simulink model "PCH_660_400_x3_6arm"  (R2018b)
settings: Solver=ode23t  StartTime=0.0  StopTime=0.1  RelTol=1e-3
undefined symbols (not defined in the file): C_load, fn, L_load, L_load1, R12pu, R_load, Rmpu, Stv, U1, U2, X12pu, Xmpu
libraries: powerlib x82, powerlib_meascontrol x27, peRmsMeasurement x17
(part 1 of 2)
settings Model: Creator=K2  LastModifiedBy=VID Company

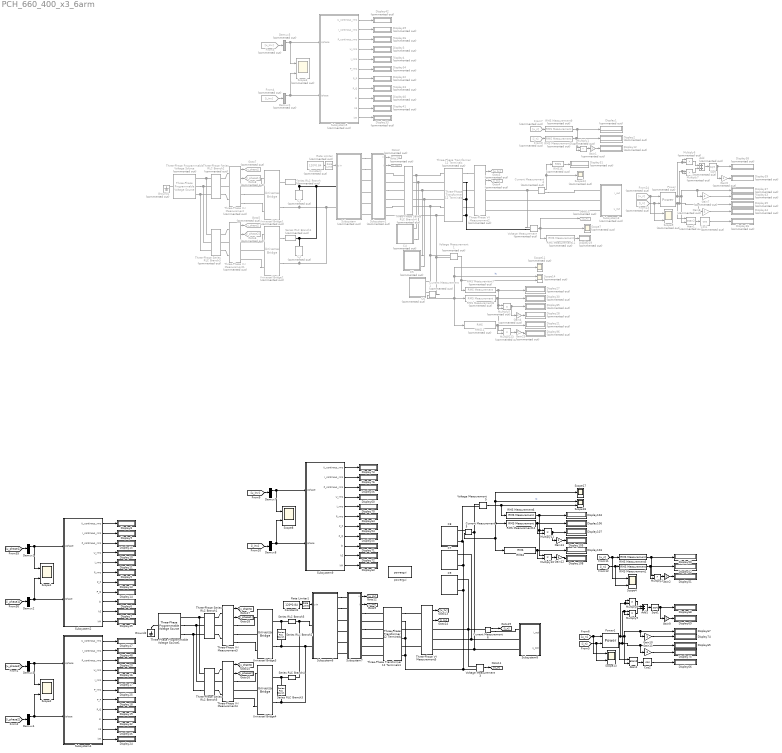
== system PCH_660_400_x3_6arm ==
  Add : Sum  Commented=on
  Add1 : Sum
  Atan1 : Trigonometry  Commented=on  Operator=atan2
  Atan2 : Trigonometry  Operator=atan2
  C4 : Subsystem  Commented=on
  C5 : Subsystem  Commented=on
  C6 : Subsystem  Commented=on
  C7 : Subsystem
  C8 : Subsystem
  C9 : Subsystem
  Constant : Constant  Commented=on  Value=120*0.84  SampleTime=1e-6
  Constant1 : Constant  Value=120*0.84  SampleTime=1e-6
  Cos1 : Trigonometry  Commented=on  Operator=cos
  Cos2 : Trigonometry  Operator=cos
  Current Measurement1 : powerlib/Measurements/Current Measurement  Commented=on  PhasorSimulation=off  OutputType=Complex  PSBequivalent=0
  Current Measurement4 : powerlib/Measurements/Current Measurement  Commented=on  PhasorSimulation=off  OutputType=Complex  PSBequivalent=0
  Current Measurement5 : powerlib/Measurements/Current Measurement  PhasorSimulation=off  OutputType=Complex  PSBequivalent=0
  Current Measurement6 : powerlib/Measurements/Current Measurement  PhasorSimulation=off  OutputType=Complex  PSBequivalent=0
  Demux{1..4,7..8} (6 alike) : Demux  Outputs=3
  Demux5 : Demux  Commented=on  Outputs=3
  Demux6 : Demux  Commented=on  Outputs=3
  Display{1..4,12,21..23,26..31,33..44,49,85,96} (29 alike) : Display  Commented=on
  Display{5..11,13..20,24..25,32,45..48,50..52,54..56,60,63..76,103..108} (49 alike) : Display
  From23 : From  Commented=on  GotoTag=i_n
  From24 : From  Commented=on  GotoTag=u_n
  From3 : From  Commented=on  GotoTag=u_inv
  From4 : From  Commented=on  GotoTag=i_inv
  From7 : From  Commented=on  GotoTag=u_n
  From8 : From  Commented=on  GotoTag=i_n
  Gain{1,4..5,7..8,23} (6 alike) : Gain  Commented=on  Gain=3
  Gain{2,9..13} (6 alike) : Gain  Gain=3
  Goto1 : Goto  Commented=on  GotoTag=i_inv
  Goto10 : Goto  Commented=on  GotoTag=u_n
  Goto2 : Goto  Commented=on  GotoTag=u_inv
  Goto3 : Goto  Commented=on  GotoTag=u_tv
  Goto4 : Goto  Commented=on  GotoTag=i_tv
  Goto5 : Goto  Commented=on  GotoTag=u_phase2
  Goto6 : Goto  Commented=on  GotoTag=i_phase2
  Goto7 : Goto  Commented=on  GotoTag=u_phase1
  Goto8 : Goto  Commented=on  GotoTag=i_phase1
  Ground1 : powerlib/Elements/Ground  Commented=on  LConnTagsString=a
  Ground2 : powerlib/Elements/Ground  LConnTagsString=a
  Multiply{1,5..7,23} (5 alike) : Product  Commented=on
  Multiply{2,8..11} (5 alike) : Product
  Power : powerlib_meascontrol/Measurements/Power  Commented=on  Freq=400  Vinit=[1, 0]  Iinit=[1, 0]  Ts=0
      settings: SourceProductName=Simscape Power Systems
  Power1 : powerlib_meascontrol/Measurements/Power  Freq=400  Vinit=[1, 0]  Iinit=[1, 0]  Ts=0
      settings: SourceProductName=Simscape Power Systems
  RMS Measurement{1,5..6,12} (4 alike) : peRmsMeasurement/RMS Measurement  LabelModeActiveChoice=Harmonic  F=400  SpecifyHarmonics=on  K=[1]  Ts=0
  RMS Measurement{7..11} (5 alike) : peRmsMeasurement/RMS Measurement  Commented=on  LabelModeActiveChoice=Harmonic  F=400  SpecifyHarmonics=on  K=[1]  Ts=0
  RMS11 : powerlib_meascontrol/Measurements/RMS  Commented=on  TrueRMS=on  Freq=400  RMSInit=0  Ts=0
  RMS16 : powerlib_meascontrol/Measurements/RMS  Commented=on  TrueRMS=on  Freq=400  RMSInit=0  Ts=0
  RMS3 : powerlib_meascontrol/Measurements/RMS  TrueRMS=on  Freq=400  RMSInit=0  Ts=0
  Rate Limiter : RateLimiter  Commented=on  RisingSlewLimit=50000  FallingSlewLimit=-50000  SampleTimeMode=inherited
  Rate Limiter1 : RateLimiter  RisingSlewLimit=50000  FallingSlewLimit=-50000  SampleTimeMode=inherited
  Scope{1..2,4,8,13,18} (6 alike) : Scope  NumInputPorts=2
  Scope11 : Scope  Commented=on
  Scope12 : Scope  Commented=on
  Scope14 : Scope  Commented=on  NumInputPorts=2
  Scope17 : Scope
  Scope3 : Scope  Commented=on  NumInputPorts=2
  Scope7 : Scope  Commented=on
  Scope9 : Scope  Commented=on  NumInputPorts=2
  Series RLC Branch : powerlib/Elements/Series RLC Branch  Commented=on  LConnTagsString=__new0  RConnTagsString=__new0  BranchType=R  Resistance=0.001  Inductance=1e-3  SetiL0=off  InitialCurrent=0  Capacitance=C_load  Setx0=off  InitialVoltage=0  Measurements=None
  Series RLC Branch1 : powerlib/Elements/Series RLC Branch  Commented=on  LConnTagsString=__new0  RConnTagsString=__new0  BranchType=R  Resistance=0.001  Inductance=1e-3  SetiL0=off  InitialCurrent=0  Capacitance=C_load  Setx0=off  InitialVoltage=0  Measurements=None
  Series RLC Branch2 : powerlib/Elements/Series RLC Branch  LConnTagsString=__new0  RConnTagsString=__new0  BranchType=C  Resistance=1  Inductance=1e-3  SetiL0=off  InitialCurrent=0  Capacitance=4500e-6  Setx0=on  InitialVoltage=909  Measurements=None
  Series RLC Branch3 : powerlib/Elements/Series RLC Branch  LConnTagsString=__new0  RConnTagsString=__new0  BranchType=C  Resistance=1  Inductance=1e-3  SetiL0=off  InitialCurrent=0  Capacitance=4500e-6  Setx0=on  InitialVoltage=910  Measurements=None
  Series RLC Branch4 : powerlib/Elements/Series RLC Branch  LConnTagsString=__new0  RConnTagsString=__new0  BranchType=R  Resistance=0.001  Inductance=1e-3  SetiL0=off  InitialCurrent=0  Capacitance=4500e-6  Setx0=on  InitialVoltage=909  Measurements=None
  Series RLC Branch5 : powerlib/Elements/Series RLC Branch  LConnTagsString=__new0  RConnTagsString=__new0  BranchType=R  Resistance=0.001  Inductance=1e-3  SetiL0=off  InitialCurrent=0  Capacitance=4500e-6  Setx0=on  InitialVoltage=909  Measurements=None
  Sqrt : Sqrt  Commented=on  SaturateOnIntegerOverflow=on
  Sqrt1 : Sqrt  SaturateOnIntegerOverflow=on
  Subsystem : Subsystem  Commented=on
  Subsystem1 : Subsystem  Commented=on
  Subsystem2 : Subsystem
  Subsystem3 : Subsystem  Commented=on
  Subsystem4 : Subsystem
  Subsystem5 : Subsystem  Commented=on
  Subsystem6 : Subsystem
  Subsystem7 : Subsystem
  Subsystem8 : Subsystem
  Subsystem9 : Subsystem
  Three-Phase Programmable Voltage Source : powerlib/Electrical Sources/Three-Phase Programmable Voltage Source  Commented=on  PositiveSequence=[690 0 50]  VariationEntity=None  VariationType=Table of time-amplitude pairs  VariationTypeAlt=Step  VariationStep=0.5  VariationRate=10  VariationMagnitude=0.3  VariationFrequency=2  VariationTiming=[1 2]  VariationPhaseA=off  Amplitudes=[1 0.8 1.2 1.0]  TimeValues=[0 0.1 0.15 0.2]  HarmonicGeneration=off  HarmonicA=[3 0.2 -25 0]  HarmonicB=[2 0.15 35 2]  Timing="[0.05  3]"  BusType=swing  Pref=0  Qref=0  Qmin=-inf  Qmax=inf
  Three-Phase Programmable Voltage Source1 : powerlib/Electrical Sources/Three-Phase Programmable Voltage Source  PositiveSequence=[690 0 50]  VariationEntity=None  VariationType=Table of time-amplitude pairs  VariationTypeAlt=Step  VariationStep=0.5  VariationRate=10  VariationMagnitude=0.3  VariationFrequency=2  VariationTiming=[1 2]  VariationPhaseA=off  Amplitudes=[1 0.8 1.2 1.0]  TimeValues=[0 0.1 0.15 0.2]  HarmonicGeneration=off  HarmonicA=[3 0.2 -25 0]  HarmonicB=[2 0.15 35 2]  Timing="[0.05  3]"  BusType=swing  Pref=0  Qref=0  Qmin=-inf  Qmax=inf
  Three-Phase Series RLC Branch1 : powerlib/Elements/Three-Phase Series RLC Branch  LConnTagsString=A|B|C  RConnTagsString=A|B|C  BranchType=L  Resistance=1  Inductance=470e-6  Capacitance=1e-6  Measurements=None
  Three-Phase Series RLC Branch2 : powerlib/Elements/Three-Phase Series RLC Branch  Commented=on  LConnTagsString=A|B|C  RConnTagsString=A|B|C  BranchType=L  Resistance=1  Inductance=470e-6  Capacitance=1e-6  Measurements=None
  Three-Phase Series RLC Branch3 : powerlib/Elements/Three-Phase Series RLC Branch  Commented=on  LConnTagsString=A|B|C  RConnTagsString=A|B|C  BranchType=L  Resistance=1  Inductance=470e-6  Capacitance=1e-6  Measurements=None
  Three-Phase Series RLC Branch4 : powerlib/Elements/Three-Phase Series RLC Branch  Commented=on  LConnTagsString=A|B|C  RConnTagsString=A|B|C  BranchType=L  Resistance=1  Inductance=L_load1  Capacitance=1e-6  Measurements=None
  Three-Phase Series RLC Branch5 : powerlib/Elements/Three-Phase Series RLC Branch  LConnTagsString=A|B|C  RConnTagsString=A|B|C  BranchType=L  Resistance=1  Inductance=470e-6  Capacitance=1e-6  Measurements=None
  Three-Phase V-I Measurement : powerlib/Measurements/Three-Phase V-I Measurement  Commented=on  VoltageMeasurement=phase-to-ground  SetLabelV=off  LabelV=Vabc  Vpu=off  VpuLL=off  CurrentMeasurement=yes  SetLabelI=off  LabelI=Iabc  Ipu=off  Pbase=100e6  Vbase=500e3  OutputType=Complex  PhasorSimulation=off  PSBequivalent=0
  Three-Phase V-I Measurement1 : powerlib/Measurements/Three-Phase V-I Measurement  Commented=on  VoltageMeasurement=phase-to-ground  SetLabelV=off  LabelV=Vabc  Vpu=off  VpuLL=off  CurrentMeasurement=yes  SetLabelI=off  LabelI=Iabc  Ipu=off  Pbase=100e6  Vbase=500e3  OutputType=Complex  PhasorSimulation=off  PSBequivalent=0
  Three-Phase V-I Measurement2 : powerlib/Measurements/Three-Phase V-I Measurement  Commented=on  VoltageMeasurement=phase-to-phase  SetLabelV=off  LabelV=Vabc  Vpu=off  VpuLL=off  CurrentMeasurement=yes  SetLabelI=off  LabelI=Iabc  Ipu=off  Pbase=100e6  Vbase=500e3  OutputType=Complex  PhasorSimulation=off  PSBequivalent=0
  Three-Phase V-I Measurement3 : powerlib/Measurements/Three-Phase V-I Measurement  VoltageMeasurement=phase-to-ground  SetLabelV=off  LabelV=Vabc  Vpu=off  VpuLL=off  CurrentMeasurement=yes  SetLabelI=off  LabelI=Iabc  Ipu=off  Pbase=100e6  Vbase=500e3  OutputType=Complex  PhasorSimulation=off  PSBequivalent=0
  Three-Phase V-I Measurement4 : powerlib/Measurements/Three-Phase V-I Measurement  VoltageMeasurement=phase-to-ground  SetLabelV=off  LabelV=Vabc  Vpu=off  VpuLL=off  CurrentMeasurement=yes  SetLabelI=off  LabelI=Iabc  Ipu=off  Pbase=100e6  Vbase=500e3  OutputType=Complex  PhasorSimulation=off  PSBequivalent=0
  Three-Phase V-I Measurement5 : powerlib/Measurements/Three-Phase V-I Measurement  VoltageMeasurement=phase-to-phase  SetLabelV=off  LabelV=Vabc  Vpu=off  VpuLL=off  CurrentMeasurement=yes  SetLabelI=off  LabelI=Iabc  Ipu=off  Pbase=100e6  Vbase=500e3  OutputType=Complex  PhasorSimulation=off  PSBequivalent=0
  Three-Phase Transformer 12 Terminals : powerlib/Elements/Three-Phase Transformer 12 Terminals  Commented=on  RatedPower=[ Stv fn ]  Winding1="[ U1 R12pu  X12pu ]"  Winding2=[ U2 R12pu X12pu]  RmXm=[ Rmpu Xmpu ]
      settings: SourceProductName=Simscape Power Systems  SourceProductBaseCode=PS
  Three-Phase Transformer 12 Terminals1 : powerlib/Elements/Three-Phase Transformer 12 Terminals  RatedPower=[ Stv fn ]  Winding1="[ U1 R12pu  X12pu ]"  Winding2=[ U2 R12pu X12pu]  RmXm=[ Rmpu Xmpu ]
      settings: SourceProductName=Simscape Power Systems  SourceProductBaseCode=PS
  Universal Bridge1 : powerlib/Power Electronics/Universal Bridge  Commented=on  Arms=3  SnubberResistance=1e5  SnubberCapacitance=inf  Device=Diodes  Ron=1e-3  Lon=0  ForwardVoltages="[  0  0  ]"  ForwardVoltage=0  GTOparameters=[ 10e-6 , 20e-6 ]  IGBTparameters=[ 1e-6 , 2e-6 ]  Measurements=None  Measurements_2=None  converterType=Rectifier
  Universal Bridge2 : powerlib/Power Electronics/Universal Bridge  Commented=on  Arms=3  SnubberResistance=1e5  SnubberCapacitance=inf  Device=Diodes  Ron=1e-3  Lon=0  ForwardVoltages="[  0  0  ]"  ForwardVoltage=0  GTOparameters=[ 10e-6 , 20e-6 ]  IGBTparameters=[ 1e-6 , 2e-6 ]  Measurements=None  Measurements_2=None  converterType=Rectifier
  Universal Bridge3 : powerlib/Power Electronics/Universal Bridge  Arms=3  SnubberResistance=1e5  SnubberCapacitance=inf  Device=Diodes  Ron=1e-3  Lon=0  ForwardVoltages="[  0  0  ]"  ForwardVoltage=0  GTOparameters=[ 10e-6 , 20e-6 ]  IGBTparameters=[ 1e-6 , 2e-6 ]  Measurements=None  Measurements_2=None  converterType=Rectifier
  Universal Bridge4 : powerlib/Power Electronics/Universal Bridge  Arms=3  SnubberResistance=1e5  SnubberCapacitance=inf  Device=Diodes  Ron=1e-3  Lon=0  ForwardVoltages="[  0  0  ]"  ForwardVoltage=0  GTOparameters=[ 10e-6 , 20e-6 ]  IGBTparameters=[ 1e-6 , 2e-6 ]  Measurements=None  Measurements_2=None  converterType=Rectifier
  Voltage Measurement : powerlib/Measurements/Voltage Measurement  Commented=on  PhasorSimulation=off  OutputType=Complex  PSBequivalent=0
  Voltage Measurement1 : powerlib/Measurements/Voltage Measurement  Commented=on  PhasorSimulation=off  OutputType=Complex  PSBequivalent=0
  Voltage Measurement3 : powerlib/Measurements/Voltage Measurement  PhasorSimulation=off  OutputType=Complex  PSBequivalent=0
  Voltage Measurement5 : powerlib/Measurements/Voltage Measurement  PhasorSimulation=off  OutputType=Complex  PSBequivalent=0
  powergui : powerlib/powergui  Priority=1  SimulationMode=Discrete  SampleTime=1e-6  frequency=60  Iterations=50  frequencyindice=0  Pbase=100e6  ErrMax=1e-4  UnitsV=kV  UnitsW=MW  buscounter=0  FunctionMessages=off  echomessages=off  EnableUseOfTLC=off  CurrentSourceSwitches=off  DisableSnubberDevices=off  DisableRonSwitches=off  DisableVfSwitches=off  DisplayEquations=off  SolverType=Tustin/Backward Euler (TBE)  Interpol=off  ExternalGateDelay=off  methode=off  Ts=100  x0status=blocks  SPID=on  SwTol=0  HookPort=off  RestoreLinks=warning  ResistiveCurrentMeasurement=off  Frange=[0:2:500]  Ylog=off  Xlog=on  ShowGrid=off  save=off  variable=ZData  structure=logsout  ZoomFFT=off  StartTime=0.007  cycles=1  DisplayStyle=1  fundamental=400  FreqAxis=off  MaxFrequency=20000  frequencyindicesteady=1  RmsSteady=1  display=off
  С1 : powerlib/Elements/Series RLC Branch  Commented=on  LConnTagsString=__new0  RConnTagsString=__new0  BranchType=C  Resistance=250*250/50e3  Inductance=1e-3  SetiL0=off  InitialCurrent=0  Capacitance=4500e-6  Setx0=on  InitialVoltage=910  Measurements=None
  С2 : powerlib/Elements/Series RLC Branch  Commented=on  LConnTagsString=__new0  RConnTagsString=__new0  BranchType=C  Resistance=250*250/50e3  Inductance=1e-3  SetiL0=off  InitialCurrent=0  Capacitance=4500e-6  Setx0=on  InitialVoltage=910  Measurements=None
  wires:
  Three-Phase V-I Measurement2/1 -> Goto3/1
  Three-Phase V-I Measurement2/2 -> Goto4/1
  Constant/1 -> Rate Limiter/1
  Rate Limiter/1 -> Subsystem/1(u in)
  Subsystem1/2(i) -> Goto1/1
  Subsystem1/1(v) -> Goto2/1
  Gain1/1 -> Display12/1
  RMS Measurement9/1 -> Display1/1, Multiply1/1
  Multiply1/1 -> Gain1/1
  RMS Measurement11/1 -> Display29/1
  Voltage Measurement/1 -> Scope7/1, Goto10/1, RMS Measurement11/1
  Current Measurement4/1 -> Scope12/1, RMS16/1
  RMS16/1 -> Display31/1
  Power/1 -> Gain7/1, Display37/1, Atan1/2, Multiply6/1, Multiply6/2
  Atan1/1 -> Cos1/1
  Cos1/1 -> Display36/1
  Power/2 -> Gain8/1, Display35/1, Multiply7/2, Multiply7/1, Atan1/1
  From24/1 -> Scope9/1, Power/1
  From23/1 -> Scope9/2, Power/2
  Multiply6/1 -> Add/1
  Multiply7/1 -> Add/2
  Add/1 -> Sqrt/1
  Sqrt/1 -> Display38/1, Gain5/1
  Gain5/1 -> Display39/1
  From7/1 -> RMS Measurement9/1
  From8/1 -> RMS Measurement10/1
  RMS Measurement10/1 -> Multiply1/2, Display2/1
  Gain7/1 -> Display43/1
  Gain8/1 -> Display44/1
  Subsystem2/10(kS) -> Display7/1
  Demux2/1 -> Scope1/2, Subsystem2/2(Iphase)
  Demux1/1 -> Scope1/1, Subsystem2/1(Uphase)
  [i_phase1] -> Demux2/1
  Subsystem2/1(U_continous_rms) -> Display8/1
  Subsystem2/11(kM) -> Display45/1
  Subsystem2/2(I_continous_rms) -> Display9/1
  Subsystem2/7(P_P) -> Display13/1
  [u_phase1] -> Demux1/1
  Subsystem2/3(P_continous_rms) -> Display15/1
  Subsystem2/8(P_Q) -> Display14/1
  Subsystem2/4(U_rms) -> Display10/1
  Subsystem2/6(P_rms) -> Display5/1
  Subsystem2/9(kI) -> Display6/1
  Subsystem2/5(I_rms) -> Display11/1
  Three-Phase V-I Measurement/1 -> Goto7/1
  Three-Phase V-I Measurement/2 -> Goto8/1
  Three-Phase V-I Measurement1/1 -> Goto5/1
  Three-Phase V-I Measurement1/2 -> Goto6/1
  Subsystem4/3(P_continous_rms) -> Display20/1
  Demux4/1 -> Subsystem4/2(Iphase), Scope2/2
  Subsystem4/2(I_continous_rms) -> Display48/1
  [i_phase2] -> Demux4/1
  Demux3/1 -> Subsystem4/1(Uphase), Scope2/1
  Subsystem4/10(kS) -> Display46/1
  Subsystem4/7(P_P) -> Display18/1
  Subsystem4/11(kM) -> Display24/1
  Subsystem4/9(kI) -> Display32/1
  Subsystem4/1(U_continous_rms) -> Display47/1
  Subsystem4/5(I_rms) -> Display17/1
  [u_phase2] -> Demux3/1
  Subsystem4/6(P_rms) -> Display25/1
  Subsystem4/8(P_Q) -> Display19/1
  Subsystem4/4(U_rms) -> Display16/1
  Subsystem5/3(P_continous_rms) -> Display26/1
  Demux6/1 -> Subsystem5/2(Iphase), Scope3/2
  Subsystem5/2(I_continous_rms) -> Display49/1
  From4/1 -> Demux6/1
  Demux5/1 -> Subsystem5/1(Uphase), Scope3/1
  Subsystem5/10(kS) -> Display41/1
  Subsystem5/7(P_P) -> Display22/1
  Subsystem5/11(kM) -> Display33/1
  Subsystem5/9(kI) -> Display40/1
  Subsystem5/1(U_continous_rms) -> Display42/1
  Subsystem5/5(I_rms) -> Display4/1
  From3/1 -> Demux5/1
  Subsystem5/6(P_rms) -> Display34/1
  Subsystem5/8(P_Q) -> Display23/1
  Subsystem5/4(U_rms) -> Display3/1
  Multiply5/1 -> Display85/1, Gain4/1
  Multiply23/1 -> Gain23/1
  Gain23/1 -> Display96/1
  RMS11/1 -> Display21/1, Multiply23/2
  Current Measurement1/1 -> RMS11/1, Scope14/1, Scope11/1, RMS Measurement8/1  "Ic"
  RMS Measurement7/1 -> Display27/1, Multiply23/1, Multiply5/1
  Gain4/1 -> Display28/1
  Voltage Measurement1/1 -> Scope14/2, RMS Measurement7/1
  RMS Measurement8/1 -> Display30/1, Multiply5/2
  Subsystem9/9(kI) -> Display71/1
  Subsystem9/6(P_rms) -> Display64/1
  Three-Phase V-I Measurement4/2 -> [i_phase2]
  Demux7/1 -> Subsystem9/1(Uphase), Scope8/1
  Subsystem9/7(P_P) -> Display54/1
  Three-Phase V-I Measurement3/2 -> [i_phase1]
  Subsystem9/1(U_continous_rms) -> Display73/1
  Gain2/1 -> Display51/1
  [u_n] -> Scope13/1, Power1/1
  Subsystem7/1(v) -> [u_inv]
  Demux8/1 -> Subsystem9/2(Iphase), Scope8/2
  Subsystem9/4(U_rms) -> Display60/1
  Add1/1 -> Sqrt1/1
  [u_inv] -> Demux7/1
  Voltage Measurement3/1 -> [u_n]
  Subsystem9/10(kS) -> Display72/1
  Subsystem9/11(kM) -> Display63/1
  Subsystem9/5(I_rms) -> Display70/1
  [i_inv] -> Demux8/1
  Gain11/1 -> Display75/1
  Subsystem9/3(P_continous_rms) -> Display56/1
  Subsystem9/2(I_continous_rms) -> Display76/1
  RMS Measurement1/1 -> Multiply2/2, Display52/1
  Three-Phase V-I Measurement4/1 -> [u_phase2]
  Sqrt1/1 -> Display68/1, Gain9/1
  Power1/1 -> Gain10/1, Display67/1, Atan2/2, Multiply8/1, Multiply8/2
  Power1/2 -> Gain11/1, Display65/1, Multiply9/2, Multiply9/1, Atan2/1
  Subsystem9/8(P_Q) -> Display55/1
  Atan2/1 -> Cos2/1
  [i_n] -> Scope4/2, RMS Measurement1/1
  [i_n] -> Scope13/2, Power1/2
  [u_n] -> Scope4/1, RMS Measurement5/1
  Three-Phase V-I Measurement3/1 -> [u_phase1]
  Multiply9/1 -> Add1/2
  Current Measurement6/1 -> [i_n]
  Cos2/1 -> Display66/1
  Multiply8/1 -> Add1/1
  Multiply2/1 -> Gain2/1
  Gain10/1 -> Display74/1
  Rate Limiter1/1 -> Subsystem6/1(u in)
  Gain9/1 -> Display69/1
  Constant1/1 -> Rate Limiter1/1
  Three-Phase V-I Measurement5/2 -> [i_tv]
  Three-Phase V-I Measurement5/1 -> [u_tv]
  RMS Measurement5/1 -> Display50/1, Multiply2/1
  Subsystem7/2(i) -> [i_inv]
  Voltage Measurement5/1 -> Scope18/2, RMS Measurement6/1
  Gain12/1 -> Display108/1
  Multiply11/1 -> Display107/1, Gain13/1
  Current Measurement5/1 -> Scope18/1, Scope17/1, RMS Measurement12/1, RMS3/1  "Ic"
  RMS Measurement6/1 -> Display104/1, Multiply10/1, Multiply11/1
  RMS3/1 -> Display103/1, Multiply10/2
  RMS Measurement12/1 -> Display106/1, Multiply11/2
  Multiply10/1 -> Gain12/1
  Gain13/1 -> Display105/1
  connections:
  Three-Phase Series RLC Branch3/LConn2 -- Three-Phase Series RLC Branch2/LConn2 -- Three-Phase Programmable Voltage Source/RConn2
  Three-Phase Programmable Voltage Source/LConn1 -- Ground1/LConn1
  Universal Bridge2/RConn2 -- Universal Bridge1/RConn2 -- С1/RConn1 -- Subsystem/LConn2 -- С2/RConn1
  Subsystem3/LConn3 -- Three-Phase V-I Measurement2/RConn3
  Three-Phase V-I Measurement2/LConn2 -- Three-Phase Transformer 12 Terminals/RConn3
  Three-Phase Transformer 12 Terminals/RConn1 -- Three-Phase V-I Measurement2/LConn1
  Universal Bridge2/RConn1 -- Series RLC Branch1/LConn1
  Subsystem/RConn1 -- Subsystem1/LConn1
  Subsystem1/LConn3 -- Subsystem/RConn3
  Subsystem1/LConn4 -- Subsystem/RConn4
  Subsystem1/LConn5 -- Subsystem/RConn5
  Subsystem1/LConn6 -- Subsystem/RConn6
  Three-Phase V-I Measurement2/LConn3 -- Three-Phase Transformer 12 Terminals/RConn5
  Subsystem3/LConn2 -- Three-Phase V-I Measurement2/RConn2
  Three-Phase Transformer 12 Terminals/LConn6 -- Voltage Measurement1/LConn2 -- Current Measurement1/LConn1 -- Subsystem1/RConn6
  Three-Phase Series RLC Branch4/LConn1 -- Subsystem1/RConn1
  Three-Phase Programmable Voltage Source/RConn3 -- Three-Phase Series RLC Branch2/LConn3 -- Three-Phase Series RLC Branch3/LConn3
  Current Measurement4/RConn1 -- Subsystem3/LConn1
  Current Measurement4/LConn1 -- Voltage Measurement/LConn1 -- Three-Phase V-I Measurement2/RConn1
  Subsystem/RConn2 -- Subsystem1/LConn2
  Three-Phase Transformer 12 Terminals/LConn2 -- C4/LConn3 -- Subsystem1/RConn2
  Three-Phase Transformer 12 Terminals/LConn4 -- C5/LConn3 -- Subsystem1/RConn4
  Three-Phase Series RLC Branch4/RConn1 -- Three-Phase Transformer 12 Terminals/LConn1 -- C4/LConn1
  Subsystem1/RConn3 -- Three-Phase Series RLC Branch4/LConn2
  Three-Phase Series RLC Branch4/RConn2 -- C5/LConn1 -- Three-Phase Transformer 12 Terminals/LConn3
  Three-Phase Series RLC Branch4/RConn3 -- C6/LConn1 -- Voltage Measurement1/LConn1 -- Three-Phase Transformer 12 Terminals/LConn5
  Three-Phase Series RLC Branch4/LConn3 -- Subsystem1/RConn5
  Voltage Measurement/LConn2 -- Three-Phase Transformer 12 Terminals/RConn6 -- Three-Phase Transformer 12 Terminals/RConn4 -- Three-Phase Transformer 12 Terminals/RConn2
  Three-Phase Series RLC Branch2/LConn1 -- Three-Phase Series RLC Branch3/LConn1 -- Three-Phase Programmable Voltage Source/RConn1
  Three-Phase V-I Measurement/LConn2 -- Three-Phase Series RLC Branch2/RConn2
  Three-Phase Series RLC Branch2/RConn1 -- Three-Phase V-I Measurement/LConn1
  Three-Phase Series RLC Branch2/RConn3 -- Three-Phase V-I Measurement/LConn3
  Three-Phase V-I Measurement/RConn1 -- Universal Bridge1/LConn1
  Three-Phase V-I Measurement/RConn2 -- Universal Bridge1/LConn2
  Three-Phase V-I Measurement/RConn3 -- Universal Bridge1/LConn3
  Three-Phase V-I Measurement1/LConn2 -- Three-Phase Series RLC Branch3/RConn2
  Three-Phase Series RLC Branch3/RConn1 -- Three-Phase V-I Measurement1/LConn1
  Three-Phase Series RLC Branch3/RConn3 -- Three-Phase V-I Measurement1/LConn3
  Three-Phase V-I Measurement1/RConn1 -- Universal Bridge2/LConn1
  Universal Bridge2/LConn2 -- Three-Phase V-I Measurement1/RConn2
  Universal Bridge2/LConn3 -- Three-Phase V-I Measurement1/RConn3
  Series RLC Branch/LConn1 -- Universal Bridge1/RConn1
  Series RLC Branch/RConn1 -- С1/LConn1 -- Series RLC Branch1/RConn1 -- С2/LConn1 -- Subsystem/LConn1
  Current Measurement1/RConn1 -- C6/LConn3
  Three-Phase Transformer 12 Terminals1/RConn2 -- Three-Phase Transformer 12 Terminals1/RConn6 -- Voltage Measurement3/LConn2 -- C9/LConn3 -- C7/LConn3 -- C8/LConn3 -- Voltage Measurement5/LConn2 -- Three-Phase Transformer 12 Terminals1/RConn4
  Three-Phase Transformer 12 Terminals1/LConn4 -- Subsystem7/RConn4
  Series RLC Branch2/RConn1 -- Universal Bridge3/RConn2 -- Universal Bridge4/RConn2 -- Series RLC Branch3/RConn1 -- Subsystem6/LConn2
  Three-Phase Series RLC Branch5/LConn3 -- Three-Phase Programmable Voltage Source1/RConn3 -- Three-Phase Series RLC Branch1/LConn3
  Three-Phase Transformer 12 Terminals1/LConn6 -- Subsystem7/RConn6
  Current Measurement6/LConn1 -- Voltage Measurement3/LConn1 -- Three-Phase V-I Measurement5/RConn1 -- C9/LConn1
  Three-Phase Transformer 12 Terminals1/LConn2 -- Subsystem7/RConn2
  Three-Phase Programmable Voltage Source1/RConn1 -- Three-Phase Series RLC Branch1/LConn1 -- Three-Phase Series RLC Branch5/LConn1
  Three-Phase V-I Measurement4/LConn2 -- Three-Phase Series RLC Branch5/RConn2
  Subsystem8/LConn2 -- Three-Phase V-I Measurement5/RConn2 -- C7/LConn1
  Three-Phase V-I Measurement3/RConn2 -- Universal Bridge3/LConn2
  Three-Phase Series RLC Branch1/RConn3 -- Three-Phase V-I Measurement3/LConn3
  Three-Phase Series RLC Branch1/RConn1 -- Three-Phase V-I Measurement3/LConn1
  Subsystem7/LConn6 -- Subsystem6/RConn6
  Three-Phase Series RLC Branch5/RConn1 -- Three-Phase V-I Measurement4/LConn1
  Subsystem8/LConn3 -- Three-Phase V-I Measurement5/RConn3 -- Voltage Measurement5/LConn1 -- Current Measurement5/LConn1
  Three-Phase V-I Measurement4/RConn1 -- Universal Bridge4/LConn1
  Subsystem7/LConn3 -- Subsystem6/RConn3
  Three-Phase V-I Measurement3/LConn2 -- Three-Phase Series RLC Branch1/RConn2
  Universal Bridge4/LConn3 -- Three-Phase V-I Measurement4/RConn3
  Three-Phase Programmable Voltage Source1/LConn1 -- Ground2/LConn1
  Three-Phase Series RLC Branch5/RConn3 -- Three-Phase V-I Measurement4/LConn3
  Subsystem7/LConn5 -- Subsystem6/RConn5
  Universal Bridge4/LConn2 -- Three-Phase V-I Measurement4/RConn2
  Three-Phase V-I Measurement3/RConn3 -- Universal Bridge3/LConn3
  Three-Phase V-I Measurement5/LConn3 -- Three-Phase Transformer 12 Terminals1/RConn5
  Three-Phase V-I Measurement3/RConn1 -- Universal Bridge3/LConn1
  Subsystem7/LConn4 -- Subsystem6/RConn4
  Current Measurement5/RConn1 -- C8/LConn1
  Subsystem6/RConn2 -- Subsystem7/LConn2
  Subsystem7/RConn3 -- Three-Phase Transformer 12 Terminals1/LConn3
  Subsystem7/RConn1 -- Three-Phase Transformer 12 Terminals1/LConn1
  Three-Phase Transformer 12 Terminals1/LConn5 -- Subsystem7/RConn5
  Three-Phase V-I Measurement5/LConn2 -- Three-Phase Transformer 12 Terminals1/RConn3
  Subsystem6/RConn1 -- Subsystem7/LConn1
  Three-Phase Transformer 12 Terminals1/RConn1 -- Three-Phase V-I Measurement5/LConn1
  Current Measurement6/RConn1 -- Subsystem8/LConn1
  Three-Phase Series RLC Branch5/LConn2 -- Three-Phase Programmable Voltage Source1/RConn2 -- Three-Phase Series RLC Branch1/LConn2
  Series RLC Branch3/LConn1 -- Series RLC Branch4/RConn1 -- Universal Bridge4/RConn1
  Series RLC Branch2/LConn1 -- Universal Bridge3/RConn1 -- Series RLC Branch5/RConn1
  Series RLC Branch5/LConn1 -- Series RLC Branch4/LConn1 -- Subsystem6/LConn1

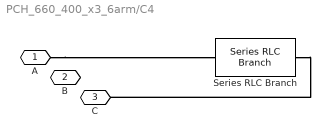
== system PCH_660_400_x3_6arm/C4 ==
  Series RLC Branch : powerlib/Elements/Series RLC Branch  LConnTagsString=__new0  RConnTagsString=__new0  BranchType=C  Resistance=1  Inductance=1e-3  SetiL0=off  InitialCurrent=0  Capacitance=C_load  Setx0=off  InitialVoltage=0  Measurements=None
  A : PMIOPort  Side=Left
  B : PMIOPort  Port=2  Side=Left
  C : PMIOPort  Port=3  Side=Left
  connections:
  Series RLC Branch/RConn1 -- C/RConn1
  A/RConn1 -- Series RLC Branch/LConn1

== system PCH_660_400_x3_6arm/C5 ==
  Series RLC Branch : powerlib/Elements/Series RLC Branch  LConnTagsString=__new0  RConnTagsString=__new0  BranchType=C  Resistance=1  Inductance=1e-3  SetiL0=off  InitialCurrent=0  Capacitance=C_load  Setx0=off  InitialVoltage=0  Measurements=None
  A : PMIOPort  Side=Left
  B : PMIOPort  Port=2  Side=Left
  C : PMIOPort  Port=3  Side=Left
  connections:
  Series RLC Branch/RConn1 -- C/RConn1
  A/RConn1 -- Series RLC Branch/LConn1

== system PCH_660_400_x3_6arm/C6 ==
  Series RLC Branch : powerlib/Elements/Series RLC Branch  LConnTagsString=__new0  RConnTagsString=__new0  BranchType=C  Resistance=1  Inductance=1e-3  SetiL0=off  InitialCurrent=0  Capacitance=C_load  Setx0=off  InitialVoltage=0  Measurements=None
  A : PMIOPort  Side=Left
  B : PMIOPort  Port=2  Side=Left
  C : PMIOPort  Port=3  Side=Left
  connections:
  Series RLC Branch/RConn1 -- C/RConn1
  A/RConn1 -- Series RLC Branch/LConn1

== system PCH_660_400_x3_6arm/C7 ==
  Series RLC Branch : powerlib/Elements/Series RLC Branch  LConnTagsString=__new0  RConnTagsString=__new0  BranchType=C  Resistance=1  Inductance=1e-3  SetiL0=off  InitialCurrent=0  Capacitance=C_load  Setx0=off  InitialVoltage=0  Measurements=None
  A : PMIOPort  Side=Left
  B : PMIOPort  Port=2  Side=Left
  C : PMIOPort  Port=3  Side=Left
  connections:
  C/RConn1 -- Series RLC Branch/RConn1
  A/RConn1 -- Series RLC Branch/LConn1

== system PCH_660_400_x3_6arm/C8 ==
  Series RLC Branch : powerlib/Elements/Series RLC Branch  LConnTagsString=__new0  RConnTagsString=__new0  BranchType=C  Resistance=1  Inductance=1e-3  SetiL0=off  InitialCurrent=0  Capacitance=C_load  Setx0=off  InitialVoltage=0  Measurements=None
  A : PMIOPort  Side=Left
  B : PMIOPort  Port=2  Side=Left
  C : PMIOPort  Port=3  Side=Left
  connections:
  Series RLC Branch/RConn1 -- C/RConn1
  A/RConn1 -- Series RLC Branch/LConn1

== system PCH_660_400_x3_6arm/C9 ==
  Series RLC Branch : powerlib/Elements/Series RLC Branch  LConnTagsString=__new0  RConnTagsString=__new0  BranchType=C  Resistance=1  Inductance=1e-3  SetiL0=off  InitialCurrent=0  Capacitance=C_load  Setx0=off  InitialVoltage=0  Measurements=None
  A : PMIOPort  Side=Left
  B : PMIOPort  Port=2  Side=Left
  C : PMIOPort  Port=3  Side=Left
  connections:
  C/RConn1 -- Series RLC Branch/RConn1
  A/RConn1 -- Series RLC Branch/LConn1

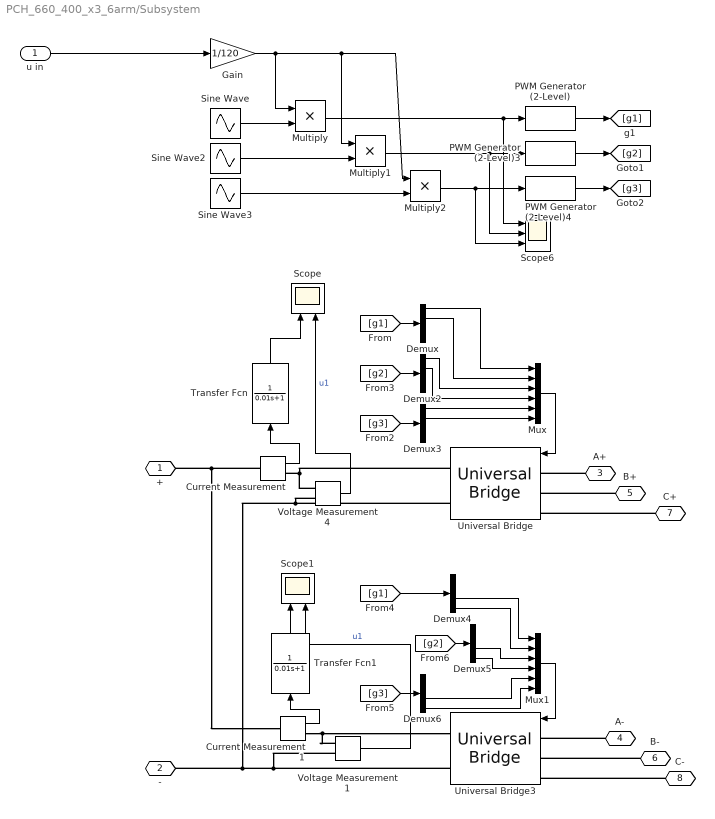
== system PCH_660_400_x3_6arm/Subsystem ==
  u in : Inport
  Current Measurement : powerlib/Measurements/Current Measurement  PhasorSimulation=off  OutputType=Complex  PSBequivalent=0
  Current Measurement1 : powerlib/Measurements/Current Measurement  PhasorSimulation=off  OutputType=Complex  PSBequivalent=0
  Demux{,2..6} (6 alike) : Demux
  Gain : Gain  Gain=1/120
  Multiply : Product
  Multiply1 : Product
  Multiply2 : Product
  Mux : Mux  Inputs=6
  Mux1 : Mux  Inputs=6
  PWM Generator (2-Level) : powerlib_meascontrol/Pulse & Signal Generators/PWM Generator (2-Level)  ModulatorType=Single-phase full-bridge (4 pulses)  ModulatorMode=Unsynchronized  Fc=fPWM  Pc=0  nF=27  MinMax="[ -1  1 ]"  SamplingTechnique=Natural  ModulatingSignals=off  m=0.8  Freq=60  Phase=0  Ts=0  ShowCarrierOutport=off
      settings: SourceProductName=Simscape Power Systems
  PWM Generator (2-Level)3 : powerlib_meascontrol/Pulse & Signal Generators/PWM Generator (2-Level)  ModulatorType=Single-phase full-bridge (4 pulses)  ModulatorMode=Unsynchronized  Fc=fPWM  Pc=120  nF=27  MinMax="[ -1  1 ]"  SamplingTechnique=Natural  ModulatingSignals=off  m=0.8  Freq=60  Phase=0  Ts=0  ShowCarrierOutport=off
      settings: SourceProductName=Simscape Power Systems
  PWM Generator (2-Level)4 : powerlib_meascontrol/Pulse & Signal Generators/PWM Generator (2-Level)  ModulatorType=Single-phase full-bridge (4 pulses)  ModulatorMode=Unsynchronized  Fc=fPWM  Pc=-120  nF=27  MinMax="[ -1  1 ]"  SamplingTechnique=Natural  ModulatingSignals=off  m=0.8  Freq=60  Phase=0  Ts=0  ShowCarrierOutport=off
      settings: SourceProductName=Simscape Power Systems
  Scope : Scope  NumInputPorts=2
  Scope1 : Scope  NumInputPorts=2
  Scope6 : Scope  NumInputPorts=3
  Sine Wave : Sin  Frequency=400*2*pi  SampleTime=0
  Sine Wave2 : Sin  Frequency=400*2*pi  Phase=-2*pi/3  SampleTime=0
  Sine Wave3 : Sin  Frequency=400*2*pi  Phase=2*pi/3  SampleTime=0
  Transfer Fcn : TransferFcn  Denominator=[0.01 1]
  Transfer Fcn1 : TransferFcn  Denominator=[0.01 1]
  Universal Bridge : powerlib/Power Electronics/Universal Bridge  Arms=3  SnubberResistance=1e5  SnubberCapacitance=inf  Device=IGBT / Diodes  Ron=5e-3  Lon=0  ForwardVoltages="[  1.5  1  ]"  ForwardVoltage=0  GTOparameters=[ 10e-6 , 20e-6 ]  IGBTparameters=[ 1e-6 , 2e-6 ]  Measurements=Device currents  Measurements_2=None  converterType=Rectifier
  Universal Bridge3 : powerlib/Power Electronics/Universal Bridge  Arms=3  SnubberResistance=1e5  SnubberCapacitance=inf  Device=IGBT / Diodes  Ron=5e-3  Lon=0  ForwardVoltages="[  1.5  1  ]"  ForwardVoltage=0  GTOparameters=[ 10e-6 , 20e-6 ]  IGBTparameters=[ 1e-6 , 2e-6 ]  Measurements=Device currents  Measurements_2=None  converterType=Rectifier
  Voltage Measurement1 : powerlib/Measurements/Voltage Measurement  PhasorSimulation=off  OutputType=Complex  PSBequivalent=0
  Voltage Measurement4 : powerlib/Measurements/Voltage Measurement  PhasorSimulation=off  OutputType=Complex  PSBequivalent=0
  + : PMIOPort  Side=Left
  - : PMIOPort  Port=2  Side=Left
  A+ : PMIOPort  Port=3  Side=Right
  A- : PMIOPort  Port=4  Side=Right
  B+ : PMIOPort  Port=5  Side=Right
  B- : PMIOPort  Port=6  Side=Right
  C+ : PMIOPort  Port=7  Side=Right
  C- : PMIOPort  Port=8  Side=Right
  wires:
  Mux1/1 -> Universal Bridge3/1
  Mux/1 -> Universal Bridge/1
  PWM Generator (2-Level)/1 -> [g1]
  Gain/1 -> Multiply2/1, Multiply1/1, Multiply/1
  u in/1 -> Gain/1
  Multiply/1 -> Scope6/1, PWM Generator (2-Level)/1
  Sine Wave/1 -> Multiply/2
  Sine Wave2/1 -> Multiply1/2
  Sine Wave3/1 -> Multiply2/2
  Multiply2/1 -> Scope6/3, PWM Generator (2-Level)4/1
  Multiply1/1 -> Scope6/2, PWM Generator (2-Level)3/1
  PWM Generator (2-Level)4/1 -> [g3]
  PWM Generator (2-Level)3/1 -> [g2]
  [g1] -> Demux/1
  Demux/1 -> Mux/1
  Demux/2 -> Mux/2
  [g2] -> Demux2/1
  Demux2/1 -> Mux/3
  Demux2/2 -> Mux/4
  [g3] -> Demux3/1
  Demux3/2 -> Mux/6
  Demux3/1 -> Mux/5
  [g1] -> Demux4/1
  Demux4/3 -> Mux1/1
  [g3] -> Demux6/1
  Demux5/4 -> Mux1/4
  Demux4/4 -> Mux1/2
  Demux5/3 -> Mux1/3
  Demux6/4 -> Mux1/6
  [g2] -> Demux5/1
  Demux6/3 -> Mux1/5
  Current Measurement/1 -> Transfer Fcn/1
  Voltage Measurement4/1 -> Scope/2  "u1"
  Voltage Measurement1/1 -> Scope1/2  "u1"
  Current Measurement1/1 -> Transfer Fcn1/1
  Transfer Fcn/1 -> Scope/1
  Transfer Fcn1/1 -> Scope1/1
  connections:
  +/RConn1 -- Current Measurement1/LConn1 -- Current Measurement/LConn1
  A+/RConn1 -- Universal Bridge/LConn1
  Universal Bridge/RConn2 -- Voltage Measurement4/LConn2 -- Universal Bridge3/RConn2 -- Voltage Measurement1/LConn2 -- -/RConn1
  B+/RConn1 -- Universal Bridge/LConn2
  C+/RConn1 -- Universal Bridge/LConn3
  C-/RConn1 -- Universal Bridge3/LConn3
  B-/RConn1 -- Universal Bridge3/LConn2
  A-/RConn1 -- Universal Bridge3/LConn1
  Voltage Measurement4/LConn1 -- Universal Bridge/RConn1 -- Current Measurement/RConn1
  Current Measurement1/RConn1 -- Universal Bridge3/RConn1 -- Voltage Measurement1/LConn1

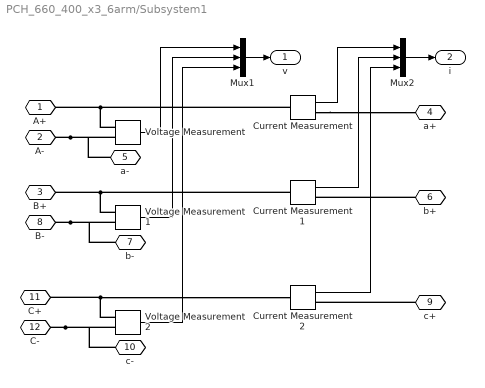
== system PCH_660_400_x3_6arm/Subsystem1 ==
  Current Measurement : powerlib/Measurements/Current Measurement  PhasorSimulation=off  OutputType=Complex  PSBequivalent=0
  Current Measurement1 : powerlib/Measurements/Current Measurement  PhasorSimulation=off  OutputType=Complex  PSBequivalent=0
  Current Measurement2 : powerlib/Measurements/Current Measurement  PhasorSimulation=off  OutputType=Complex  PSBequivalent=0
  Mux1 : Mux  Inputs=3
  Mux2 : Mux  Inputs=3
  Voltage Measurement : powerlib/Measurements/Voltage Measurement  PhasorSimulation=off  OutputType=Complex  PSBequivalent=0
  Voltage Measurement1 : powerlib/Measurements/Voltage Measurement  PhasorSimulation=off  OutputType=Complex  PSBequivalent=0
  Voltage Measurement2 : powerlib/Measurements/Voltage Measurement  PhasorSimulation=off  OutputType=Complex  PSBequivalent=0
  A+ : PMIOPort  Side=Left
  A- : PMIOPort  Port=2  Side=Left
  B+ : PMIOPort  Port=3  Side=Left
  a+ : PMIOPort  Port=4  Side=Right
  a- : PMIOPort  Port=5  Side=Right
  b+ : PMIOPort  Port=6  Side=Right
  b- : PMIOPort  Port=7  Side=Right
  B- : PMIOPort  Port=8  Side=Left
  c+ : PMIOPort  Port=9  Side=Right
  c- : PMIOPort  Port=10  Side=Right
  C+ : PMIOPort  Port=11  Side=Left
  C- : PMIOPort  Port=12  Side=Left
  v : Outport
  i : Outport  Port=2
  wires:
  Voltage Measurement1/1 -> Mux1/2
  Current Measurement2/1 -> Mux2/3
  Voltage Measurement2/1 -> Mux1/3
  Current Measurement/1 -> Mux2/1
  Voltage Measurement/1 -> Mux1/1
  Mux1/1 -> v/1
  Current Measurement1/1 -> Mux2/2
  Mux2/1 -> i/1
  connections:
  Current Measurement/RConn1 -- a+/RConn1
  Current Measurement/LConn1 -- Voltage Measurement/LConn1 -- A+/RConn1
  Voltage Measurement2/LConn1 -- Current Measurement2/LConn1 -- C+/RConn1
  c+/RConn1 -- Current Measurement2/RConn1
  Current Measurement1/LConn1 -- Voltage Measurement1/LConn1 -- B+/RConn1
  B-/RConn1 -- Voltage Measurement1/LConn2 -- b-/RConn1
  b+/RConn1 -- Current Measurement1/RConn1
  A-/RConn1 -- Voltage Measurement/LConn2 -- a-/RConn1
  C-/RConn1 -- Voltage Measurement2/LConn2 -- c-/RConn1

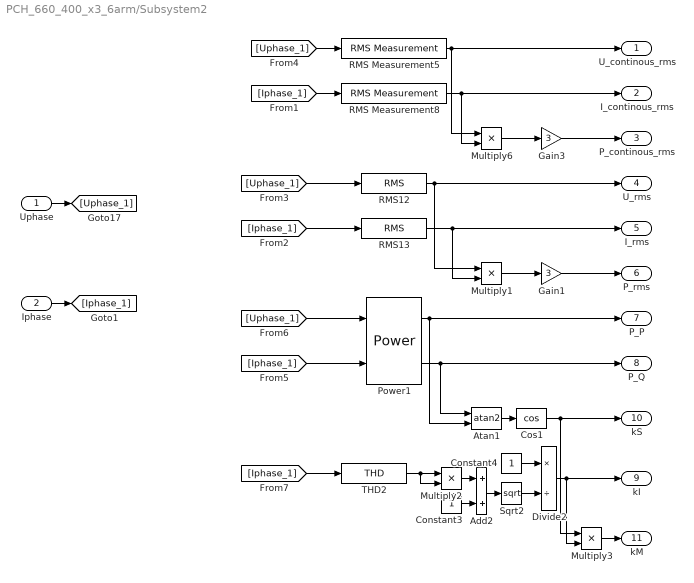
== system PCH_660_400_x3_6arm/Subsystem2 ==
  Uphase : Inport
  Iphase : Inport  Port=2
  Add2 : Sum
  Atan1 : Trigonometry  Operator=atan2
  Constant3 : Constant
  Constant4 : Constant
  Cos1 : Trigonometry  Operator=cos
  Divide2 : Product  Inputs=*/
  Gain1 : Gain  Gain=3
  Gain3 : Gain  Gain=3
  Multiply{1..3,6} (4 alike) : Product
  Power1 : powerlib_meascontrol/Measurements/Power  Freq=50  Vinit=[1, 0]  Iinit=[1, 0]  Ts=0
      settings: SourceProductName=Simscape Power Systems
  RMS Measurement5 : peRmsMeasurement/RMS Measurement  LabelModeActiveChoice=Harmonic  F=50  SpecifyHarmonics=on  K=[1]  Ts=0
  RMS Measurement8 : peRmsMeasurement/RMS Measurement  LabelModeActiveChoice=Harmonic  F=50  SpecifyHarmonics=on  K=[1]  Ts=0
  RMS12 : powerlib_meascontrol/Measurements/RMS  TrueRMS=on  Freq=50  RMSInit=0  Ts=0
  RMS13 : powerlib_meascontrol/Measurements/RMS  TrueRMS=on  Freq=50  RMSInit=0  Ts=0
  Sqrt2 : Sqrt  SaturateOnIntegerOverflow=on
  THD2 : powerlib_meascontrol/Measurements/THD  Freq=50  Ts=0
  U_continous_rms : Outport
  I_continous_rms : Outport  Port=2
  P_continous_rms : Outport  Port=3
  U_rms : Outport  Port=4
  I_rms : Outport  Port=5
  P_rms : Outport  Port=6
  P_P : Outport  Port=7
  P_Q : Outport  Port=8
  kI : Outport  Port=9
  kS : Outport  Port=10
  kM : Outport  Port=11
  wires:
  RMS Measurement5/1 -> Multiply6/1, U_continous_rms/1
  RMS Measurement8/1 -> Multiply6/2, I_continous_rms/1
  [Uphase_1] -> RMS Measurement5/1
  [Iphase_1] -> RMS Measurement8/1
  Multiply6/1 -> Gain3/1
  RMS12/1 -> Multiply1/1, U_rms/1
  [Uphase_1] -> RMS12/1
  [Iphase_1] -> RMS13/1
  RMS13/1 -> Multiply1/2, I_rms/1
  Multiply1/1 -> Gain1/1
  Atan1/1 -> Cos1/1
  Power1/1 -> Atan1/2, P_P/1
  Power1/2 -> Atan1/1, P_Q/1
  [Uphase_1] -> Power1/1
  [Iphase_1] -> Power1/2
  Cos1/1 -> Multiply3/1, kS/1
  Sqrt2/1 -> Divide2/2
  THD2/1 -> Multiply2/1, Multiply2/2
  Constant3/1 -> Add2/2
  Multiply2/1 -> Add2/1
  Constant4/1 -> Divide2/1
  Divide2/1 -> Multiply3/2, kI/1
  Add2/1 -> Sqrt2/1
  [Iphase_1] -> THD2/1
  Multiply3/1 -> kM/1
  Gain3/1 -> P_continous_rms/1
  Gain1/1 -> P_rms/1
  Uphase/1 -> [Uphase_1]
  Iphase/1 -> [Iphase_1]

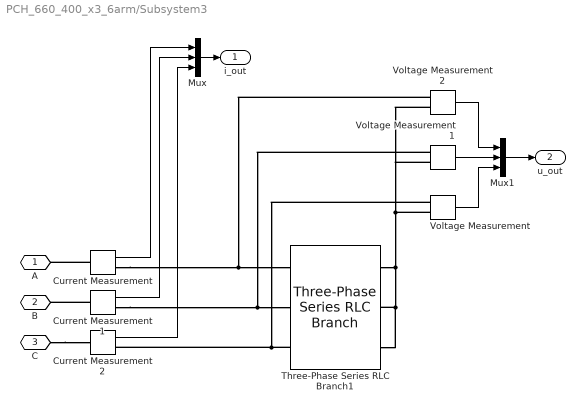
== system PCH_660_400_x3_6arm/Subsystem3 ==
  Current Measurement : powerlib/Measurements/Current Measurement  PhasorSimulation=off  OutputType=Complex  PSBequivalent=0
  Current Measurement1 : powerlib/Measurements/Current Measurement  PhasorSimulation=off  OutputType=Complex  PSBequivalent=0
  Current Measurement2 : powerlib/Measurements/Current Measurement  PhasorSimulation=off  OutputType=Complex  PSBequivalent=0
  Mux : Mux  Inputs=3
  Mux1 : Mux  Inputs=3
  Three-Phase Series RLC Branch1 : powerlib/Elements/Three-Phase Series RLC Branch  LConnTagsString=A|B|C  RConnTagsString=A|B|C  BranchType=RL  Resistance=R_load  Inductance=L_load  Capacitance=105e-6  Measurements=None
  Voltage Measurement : powerlib/Measurements/Voltage Measurement  PhasorSimulation=off  OutputType=Complex  PSBequivalent=0
  Voltage Measurement1 : powerlib/Measurements/Voltage Measurement  PhasorSimulation=off  OutputType=Complex  PSBequivalent=0
  Voltage Measurement2 : powerlib/Measurements/Voltage Measurement  PhasorSimulation=off  OutputType=Complex  PSBequivalent=0
  A : PMIOPort  Side=Left
  B : PMIOPort  Port=2  Side=Left
  C : PMIOPort  Port=3  Side=Left
  i_out : Outport
  u_out : Outport  Port=2
  wires:
  Mux/1 -> i_out/1
  Current Measurement/1 -> Mux/1
  Current Measurement1/1 -> Mux/2
  Current Measurement2/1 -> Mux/3
  Voltage Measurement1/1 -> Mux1/2
  Voltage Measurement2/1 -> Mux1/1
  Voltage Measurement/1 -> Mux1/3
  Mux1/1 -> u_out/1
  connections:
  Three-Phase Series RLC Branch1/RConn3 -- Voltage Measurement2/LConn2 -- Voltage Measurement1/LConn2 -- Voltage Measurement/LConn2 -- Three-Phase Series RLC Branch1/RConn1 -- Three-Phase Series RLC Branch1/RConn2
  Current Measurement1/LConn1 -- B/RConn1
  Current Measurement/LConn1 -- A/RConn1
  Three-Phase Series RLC Branch1/LConn3 -- Voltage Measurement/LConn1 -- Current Measurement2/RConn1
  Current Measurement/RConn1 -- Voltage Measurement2/LConn1 -- Three-Phase Series RLC Branch1/LConn1
  Current Measurement1/RConn1 -- Voltage Measurement1/LConn1 -- Three-Phase Series RLC Branch1/LConn2
  C/RConn1 -- Current Measurement2/LConn1

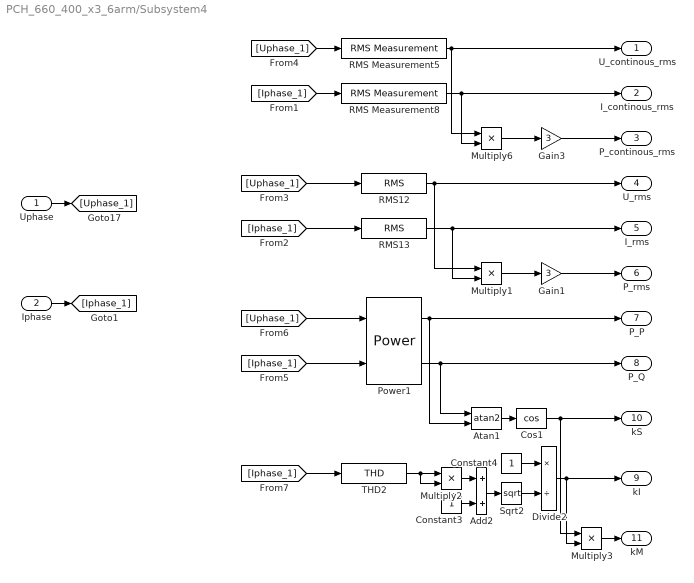
== system PCH_660_400_x3_6arm/Subsystem4 ==
  Uphase : Inport
  Iphase : Inport  Port=2
  Add2 : Sum
  Atan1 : Trigonometry  Operator=atan2
  Constant3 : Constant
  Constant4 : Constant
  Cos1 : Trigonometry  Operator=cos
  Divide2 : Product  Inputs=*/
  Gain1 : Gain  Gain=3
  Gain3 : Gain  Gain=3
  Multiply{1..3,6} (4 alike) : Product
  Power1 : powerlib_meascontrol/Measurements/Power  Freq=50  Vinit=[1, 0]  Iinit=[1, 0]  Ts=0
      settings: SourceProductName=Simscape Power Systems
  RMS Measurement5 : peRmsMeasurement/RMS Measurement  LabelModeActiveChoice=Harmonic  F=50  SpecifyHarmonics=on  K=[1]  Ts=0
  RMS Measurement8 : peRmsMeasurement/RMS Measurement  LabelModeActiveChoice=Harmonic  F=50  SpecifyHarmonics=on  K=[1]  Ts=0
  RMS12 : powerlib_meascontrol/Measurements/RMS  TrueRMS=on  Freq=50  RMSInit=0  Ts=0
  RMS13 : powerlib_meascontrol/Measurements/RMS  TrueRMS=on  Freq=50  RMSInit=0  Ts=0
  Sqrt2 : Sqrt  SaturateOnIntegerOverflow=on
  THD2 : powerlib_meascontrol/Measurements/THD  Freq=50  Ts=0
  U_continous_rms : Outport
  I_continous_rms : Outport  Port=2
  P_continous_rms : Outport  Port=3
  U_rms : Outport  Port=4
  I_rms : Outport  Port=5
  P_rms : Outport  Port=6
  P_P : Outport  Port=7
  P_Q : Outport  Port=8
  kI : Outport  Port=9
  kS : Outport  Port=10
  kM : Outport  Port=11
  wires:
  RMS Measurement5/1 -> Multiply6/1, U_continous_rms/1
  RMS Measurement8/1 -> Multiply6/2, I_continous_rms/1
  [Uphase_1] -> RMS Measurement5/1
  [Iphase_1] -> RMS Measurement8/1
  Multiply6/1 -> Gain3/1
  RMS12/1 -> Multiply1/1, U_rms/1
  [Uphase_1] -> RMS12/1
  [Iphase_1] -> RMS13/1
  RMS13/1 -> Multiply1/2, I_rms/1
  Multiply1/1 -> Gain1/1
  Atan1/1 -> Cos1/1
  Power1/1 -> Atan1/2, P_P/1
  Power1/2 -> Atan1/1, P_Q/1
  [Uphase_1] -> Power1/1
  [Iphase_1] -> Power1/2
  Cos1/1 -> Multiply3/1, kS/1
  Sqrt2/1 -> Divide2/2
  THD2/1 -> Multiply2/1, Multiply2/2
  Constant3/1 -> Add2/2
  Multiply2/1 -> Add2/1
  Constant4/1 -> Divide2/1
  Divide2/1 -> Multiply3/2, kI/1
  Add2/1 -> Sqrt2/1
  [Iphase_1] -> THD2/1
  Multiply3/1 -> kM/1
  Gain3/1 -> P_continous_rms/1
  Gain1/1 -> P_rms/1
  Uphase/1 -> [Uphase_1]
  Iphase/1 -> [Iphase_1]

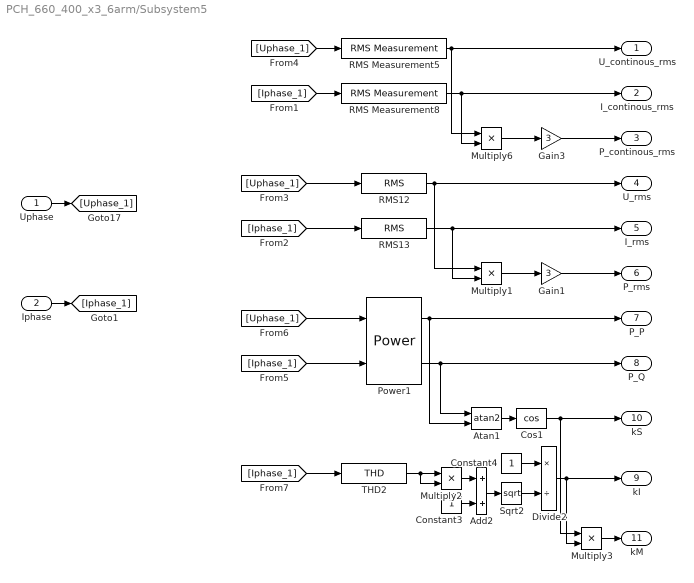
== system PCH_660_400_x3_6arm/Subsystem5 ==
  Uphase : Inport
  Iphase : Inport  Port=2
  Add2 : Sum
  Atan1 : Trigonometry  Operator=atan2
  Constant3 : Constant
  Constant4 : Constant
  Cos1 : Trigonometry  Operator=cos
  Divide2 : Product  Inputs=*/
  Gain1 : Gain  Gain=3
  Gain3 : Gain  Gain=3
  Multiply{1..3,6} (4 alike) : Product
  Power1 : powerlib_meascontrol/Measurements/Power  Freq=400  Vinit=[1, 0]  Iinit=[1, 0]  Ts=0
      settings: SourceProductName=Simscape Power Systems
  RMS Measurement5 : peRmsMeasurement/RMS Measurement  LabelModeActiveChoice=Harmonic  F=400  SpecifyHarmonics=on  K=[1]  Ts=0
  RMS Measurement8 : peRmsMeasurement/RMS Measurement  LabelModeActiveChoice=Harmonic  F=400  SpecifyHarmonics=on  K=[1]  Ts=0
  RMS12 : powerlib_meascontrol/Measurements/RMS  TrueRMS=on  Freq=400  RMSInit=0  Ts=0
  RMS13 : powerlib_meascontrol/Measurements/RMS  TrueRMS=on  Freq=400  RMSInit=0  Ts=0
  Sqrt2 : Sqrt  SaturateOnIntegerOverflow=on
  THD2 : powerlib_meascontrol/Measurements/THD  Freq=400  Ts=0
  U_continous_rms : Outport
  I_continous_rms : Outport  Port=2
  P_continous_rms : Outport  Port=3
  U_rms : Outport  Port=4
  I_rms : Outport  Port=5
  P_rms : Outport  Port=6
  P_P : Outport  Port=7
  P_Q : Outport  Port=8
  kI : Outport  Port=9
  kS : Outport  Port=10
  kM : Outport  Port=11
  wires:
  RMS Measurement5/1 -> Multiply6/1, U_continous_rms/1
  RMS Measurement8/1 -> Multiply6/2, I_continous_rms/1
  [Uphase_1] -> RMS Measurement5/1
  [Iphase_1] -> RMS Measurement8/1
  Multiply6/1 -> Gain3/1
  RMS12/1 -> Multiply1/1, U_rms/1
  [Uphase_1] -> RMS12/1
  [Iphase_1] -> RMS13/1
  RMS13/1 -> Multiply1/2, I_rms/1
  Multiply1/1 -> Gain1/1
  Atan1/1 -> Cos1/1
  Power1/1 -> Atan1/2, P_P/1
  Power1/2 -> Atan1/1, P_Q/1
  [Uphase_1] -> Power1/1
  [Iphase_1] -> Power1/2
  Cos1/1 -> Multiply3/1, kS/1
  Sqrt2/1 -> Divide2/2
  THD2/1 -> Multiply2/1, Multiply2/2
  Constant3/1 -> Add2/2
  Multiply2/1 -> Add2/1
  Constant4/1 -> Divide2/1
  Divide2/1 -> Multiply3/2, kI/1
  Add2/1 -> Sqrt2/1
  [Iphase_1] -> THD2/1
  Multiply3/1 -> kM/1
  Gain3/1 -> P_continous_rms/1
  Gain1/1 -> P_rms/1
  Uphase/1 -> [Uphase_1]
  Iphase/1 -> [Iphase_1]

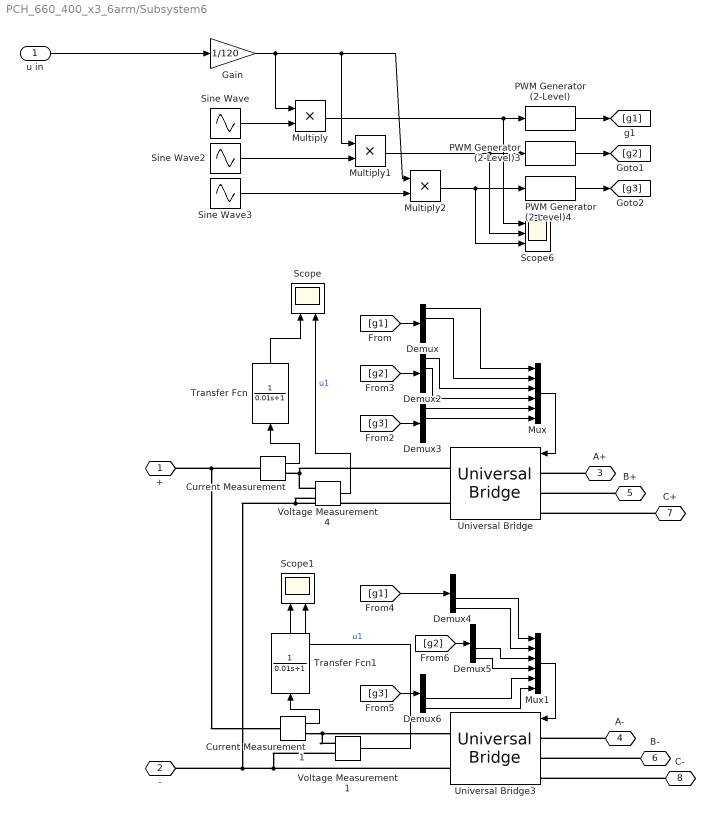
== system PCH_660_400_x3_6arm/Subsystem6 ==
  u in : Inport
  Current Measurement : powerlib/Measurements/Current Measurement  PhasorSimulation=off  OutputType=Complex  PSBequivalent=0
  Current Measurement1 : powerlib/Measurements/Current Measurement  PhasorSimulation=off  OutputType=Complex  PSBequivalent=0
  Demux{,2..6} (6 alike) : Demux
  Gain : Gain  Gain=1/120
  Multiply : Product
  Multiply1 : Product
  Multiply2 : Product
  Mux : Mux  Inputs=6
  Mux1 : Mux  Inputs=6
  PWM Generator (2-Level) : powerlib_meascontrol/Pulse & Signal Generators/PWM Generator (2-Level)  ModulatorType=Single-phase full-bridge (4 pulses)  ModulatorMode=Unsynchronized  Fc=fPWM  Pc=0  nF=27  MinMax="[ -1  1 ]"  SamplingTechnique=Natural  ModulatingSignals=off  m=0.8  Freq=60  Phase=0  Ts=0  ShowCarrierOutport=off
      settings: SourceProductName=Simscape Power Systems
  PWM Generator (2-Level)3 : powerlib_meascontrol/Pulse & Signal Generators/PWM Generator (2-Level)  ModulatorType=Single-phase full-bridge (4 pulses)  ModulatorMode=Unsynchronized  Fc=fPWM  Pc=120  nF=27  MinMax="[ -1  1 ]"  SamplingTechnique=Natural  ModulatingSignals=off  m=0.8  Freq=60  Phase=0  Ts=0  ShowCarrierOutport=off
      settings: SourceProductName=Simscape Power Systems
  PWM Generator (2-Level)4 : powerlib_meascontrol/Pulse & Signal Generators/PWM Generator (2-Level)  ModulatorType=Single-phase full-bridge (4 pulses)  ModulatorMode=Unsynchronized  Fc=fPWM  Pc=-120  nF=27  MinMax="[ -1  1 ]"  SamplingTechnique=Natural  ModulatingSignals=off  m=0.8  Freq=60  Phase=0  Ts=0  ShowCarrierOutport=off
      settings: SourceProductName=Simscape Power Systems
  Scope : Scope  NumInputPorts=2
  Scope1 : Scope  NumInputPorts=2
  Scope6 : Scope  NumInputPorts=3
  Sine Wave : Sin  Frequency=400*2*pi  SampleTime=0
  Sine Wave2 : Sin  Frequency=400*2*pi  Phase=-2*pi/3  SampleTime=0
  Sine Wave3 : Sin  Frequency=400*2*pi  Phase=2*pi/3  SampleTime=0
  Transfer Fcn : TransferFcn  Denominator=[0.01 1]
  Transfer Fcn1 : TransferFcn  Denominator=[0.01 1]
  Universal Bridge : powerlib/Power Electronics/Universal Bridge  Arms=3  SnubberResistance=1e5  SnubberCapacitance=inf  Device=IGBT / Diodes  Ron=5e-3  Lon=0  ForwardVoltages="[  1.5  1  ]"  ForwardVoltage=0  GTOparameters=[ 10e-6 , 20e-6 ]  IGBTparameters=[ 1e-6 , 2e-6 ]  Measurements=Device currents  Measurements_2=None  converterType=Rectifier
  Universal Bridge3 : powerlib/Power Electronics/Universal Bridge  Arms=3  SnubberResistance=1e5  SnubberCapacitance=inf  Device=IGBT / Diodes  Ron=5e-3  Lon=0  ForwardVoltages="[  1.5  1  ]"  ForwardVoltage=0  GTOparameters=[ 10e-6 , 20e-6 ]  IGBTparameters=[ 1e-6 , 2e-6 ]  Measurements=Device currents  Measurements_2=None  converterType=Rectifier
  Voltage Measurement1 : powerlib/Measurements/Voltage Measurement  PhasorSimulation=off  OutputType=Complex  PSBequivalent=0
  Voltage Measurement4 : powerlib/Measurements/Voltage Measurement  PhasorSimulation=off  OutputType=Complex  PSBequivalent=0
  + : PMIOPort  Side=Left
  - : PMIOPort  Port=2  Side=Left
  A+ : PMIOPort  Port=3  Side=Right
  A- : PMIOPort  Port=4  Side=Right
  B+ : PMIOPort  Port=5  Side=Right
  B- : PMIOPort  Port=6  Side=Right
  C+ : PMIOPort  Port=7  Side=Right
  C- : PMIOPort  Port=8  Side=Right
  wires:
  Mux1/1 -> Universal Bridge3/1
  Mux/1 -> Universal Bridge/1
  PWM Generator (2-Level)/1 -> [g1]
  Gain/1 -> Multiply2/1, Multiply1/1, Multiply/1
  u in/1 -> Gain/1
  Multiply/1 -> Scope6/1, PWM Generator (2-Level)/1
  Sine Wave/1 -> Multiply/2
  Sine Wave2/1 -> Multiply1/2
  Sine Wave3/1 -> Multiply2/2
  Multiply2/1 -> Scope6/3, PWM Generator (2-Level)4/1
  Multiply1/1 -> Scope6/2, PWM Generator (2-Level)3/1
  PWM Generator (2-Level)4/1 -> [g3]
  PWM Generator (2-Level)3/1 -> [g2]
  [g1] -> Demux/1
  Demux/1 -> Mux/1
  Demux/2 -> Mux/2
  [g2] -> Demux2/1
  Demux2/1 -> Mux/3
  Demux2/2 -> Mux/4
  [g3] -> Demux3/1
  Demux3/2 -> Mux/6
  Demux3/1 -> Mux/5
  [g1] -> Demux4/1
  Demux4/3 -> Mux1/1
  [g3] -> Demux6/1
  Demux5/4 -> Mux1/4
  Demux4/4 -> Mux1/2
  Demux5/3 -> Mux1/3
  Demux6/4 -> Mux1/6
  [g2] -> Demux5/1
  Demux6/3 -> Mux1/5
  Current Measurement/1 -> Transfer Fcn/1
  Voltage Measurement4/1 -> Scope/2  "u1"
  Voltage Measurement1/1 -> Scope1/2  "u1"
  Current Measurement1/1 -> Transfer Fcn1/1
  Transfer Fcn/1 -> Scope/1
  Transfer Fcn1/1 -> Scope1/1
  connections:
  +/RConn1 -- Current Measurement1/LConn1 -- Current Measurement/LConn1
  A+/RConn1 -- Universal Bridge/LConn1
  Universal Bridge/RConn2 -- Voltage Measurement4/LConn2 -- Universal Bridge3/RConn2 -- Voltage Measurement1/LConn2 -- -/RConn1
  B+/RConn1 -- Universal Bridge/LConn2
  C+/RConn1 -- Universal Bridge/LConn3
  C-/RConn1 -- Universal Bridge3/LConn3
  B-/RConn1 -- Universal Bridge3/LConn2
  A-/RConn1 -- Universal Bridge3/LConn1
  Voltage Measurement4/LConn1 -- Universal Bridge/RConn1 -- Current Measurement/RConn1
  Current Measurement1/RConn1 -- Universal Bridge3/RConn1 -- Voltage Measurement1/LConn1
